simulink model "simulation"  (R2023b)
settings: Solver=VariableStepAuto  StartTime=0.0  StopTime=10.0  RelTol=1e-3
values from neighbouring files (symbols this model uses):
  b1 = b(1,:)    [main.m]    (also in sam_model.m)
  b2 = b(2,:)    [main.m]    (also in sam_model.m)
undefined symbols (not defined in the file or in its folder): a
libraries: fuzblock x2
settings Model: Creator=samee  LastModifiedBy=srd2

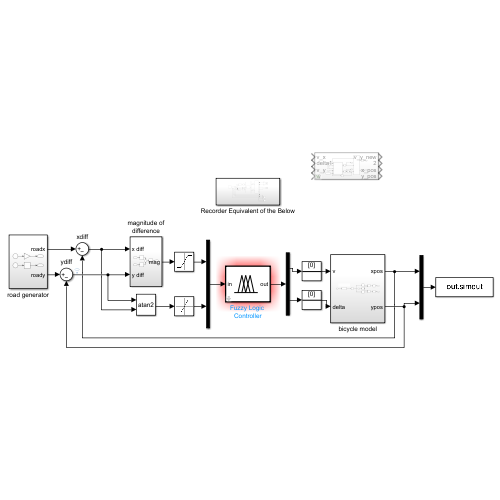
[thumbnail: Simulink's stored preview of the top-level diagram]
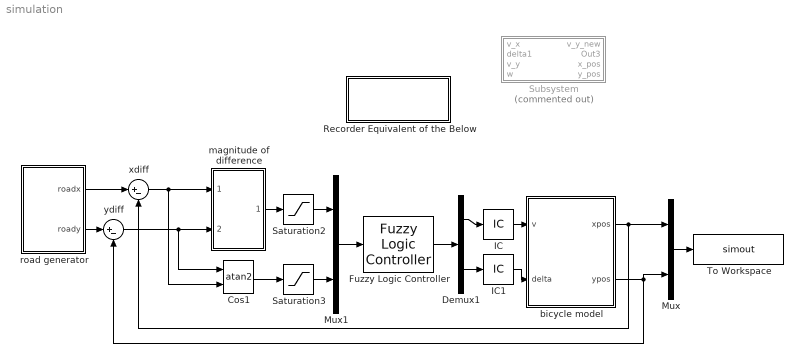
== system simulation ==
  Cos1 : Trigonometry  Operator=atan2
  Demux1 : Demux  Outputs=2
  Fuzzy Logic Controller : fuzblock/Fuzzy Logic  Controller  FIS=fis  OutputSampleNumber=101  DataType=double  FuzzifiedInputs=off  RuleFiringStrengths=off  RuleOutputs=off  AggregatedOutputs=off  SimulateUsing=Interpreted execution  OutOfRangeInputValueMessage=warning  NoRuleFiredMessage=warning  EmptyOutputFuzzySetMessage=warning
  IC : InitialCondition  Value=0
  IC1 : InitialCondition  Value=0
  Mux : Mux  Inputs=2
  Mux1 : Mux  Inputs=2
  Recorder Equivalent of the Below : Subsystem
  Saturation2 : Saturate  UpperLimit=5  LowerLimit=0  LinearizeAsGain=off
  Saturation3 : Saturate  UpperLimit=1  LowerLimit=-1
  Subsystem : Subsystem  Commented=on
  To Workspace : ToWorkspace  VariableName=simout  SaveFormat=Timeseries  SampleTime=-1
  bicycle model : Subsystem
  magnitude of difference : Subsystem
  road generator : Subsystem
  xdiff : Sum  Inputs=|+-
  ydiff : Sum  Inputs=|+-
  wires:
  Saturation2/1 -> Mux1/1
  Fuzzy Logic Controller/1 -> Demux1/1
  Demux1/2 -> IC1/1
  ydiff/1 -> Cos1/1, magnitude of difference/2(y diff)
  Mux1/1 -> Fuzzy Logic Controller/1
  road generator/2(roady) -> ydiff/1
  road generator/1(roadx) -> xdiff/1
  Demux1/1 -> IC/1
  IC1/1 -> bicycle model/2(delta)
  magnitude of difference/1(mag) -> Saturation2/1
  Saturation3/1 -> Mux1/2
  bicycle model/1(xpos) -> Mux/1, xdiff/2
  Cos1/1 -> Saturation3/1
  xdiff/1 -> Cos1/2, magnitude of difference/1(x diff)
  IC/1 -> bicycle model/1(v)
  bicycle model/2(ypos) -> Mux/2, ydiff/2
  Mux/1 -> To Workspace/1

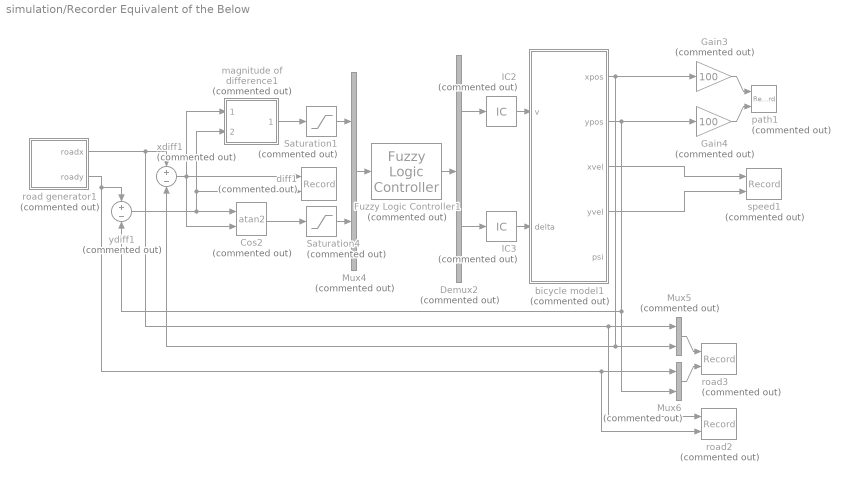
== system simulation/Recorder Equivalent of the Below ==
  Cos2 : Trigonometry  Commented=on  Operator=atan2
  Demux2 : Demux  Commented=on  Outputs=2
  Fuzzy Logic Controller1 : fuzblock/Fuzzy Logic  Controller  Commented=on  FIS=fis  OutputSampleNumber=101  DataType=double  FuzzifiedInputs=off  RuleFiringStrengths=off  RuleOutputs=off  AggregatedOutputs=off  SimulateUsing=Interpreted execution  OutOfRangeInputValueMessage=warning  NoRuleFiredMessage=warning  EmptyOutputFuzzySetMessage=warning
  Gain3 : Gain  Commented=on  Gain=100
  Gain4 : Gain  Commented=on  Gain=100
  IC2 : InitialCondition  Commented=on  Value=0
  IC3 : InitialCondition  Commented=on  Value=0
  Mux4 : Mux  Commented=on  Inputs=2
  Mux5 : Mux  Commented=on  Inputs=2
  Mux6 : Mux  Commented=on  Inputs=2
  Saturation1 : Saturate  Commented=on  UpperLimit=100  LowerLimit=0  LinearizeAsGain=off
  Saturation4 : Saturate  Commented=on  UpperLimit=1  LowerLimit=-1
  bicycle model1 : Subsystem  Commented=on
  diff1 : Record  Commented=on  FileSettingsInternal="{\"entries\":[{\"content\":{\"excelSettings\":{\"content\":{},\"type\":\"Streamout.ExcelSettings\"}},\"type\":\"Streamout.FileSettingStorage\",\"uuid\":\"\"}],\"packageUris\":[\"http:\\/\\/schema.mathworks.com\\/mf0\\/streamout_blocks\\/R2020a\"],\"version\":\"1.0\"}"  Layout=[1 1]  SignalsInternal="{\"entries\":[{\"content\":{\"signals\":[{\"content\":{\"blockPath\":[],\"dimensions\":[1],\"domain\":\"\",\"lineColor\":\"#edb120\",\"plots\":[1],\"port\":1,\"signalID\":48,\"signalName\":\"xdiff\"},\"type\":\"RecordBlkView.Signal\",\"uuid\":\"\"},{\"content\":{\"blockPath\":[],\"dimensions\":[1],\"domain\":\"\",\"lineColor\":\"#7e2f8e\",\"plots\":[1],\"port\":2,\"signalID\":51,\"signalName\":\"ydiff\"},\"type\":\"RecordBlkView.Signal\",\"uuid\":\"\"}]},\"type\":\"RecordBlkView.InputSignals\",\"uuid\":\"\"}],\"packageUris\":[\"http:\\/\\/schema.mathworks.com\\/mf0\\/streamout_blocks\\/R2020a\"],\"version\":\"1.0\"}"  VisualizationBindings="{\"xyplotplugin\":{\"info\":[{\"series\":[{\"bindingParametersList\":[{\"parameter\":\"X-Axis\",\"signalID\":48,\"signalName\":\"xdiff\"},{\"parameter\":\"Y-Axis\",\"signalID\":51,\"signalName\":\"ydiff\"}],\"seriesID\":23733}],\"subplotID\":1}]}}"  CompatibilityTag=XY
  magnitude of difference1 : Subsystem  Commented=on
  path1 : Record  Commented=on  FileSettingsInternal="{\"entries\":[{\"content\":{\"excelSettings\":{\"content\":{},\"type\":\"Streamout.ExcelSettings\"}},\"type\":\"Streamout.FileSettingStorage\",\"uuid\":\"\"}],\"packageUris\":[\"http:\\/\\/schema.mathworks.com\\/mf0\\/streamout_blocks\\/R2020a\"],\"version\":\"1.0\"}"  Layout=[1 1]  SignalsInternal="{\"entries\":[{\"content\":{\"signals\":[{\"content\":{\"blockPath\":[],\"dimensions\":[1],\"domain\":\"\",\"lineColor\":\"#77ac30\",\"plots\":[1],\"port\":1,\"signalID\":40,\"signalName\":\"Gain\"},\"type\":\"RecordBlkView.Signal\",\"uuid\":\"\"},{\"content\":{\"blockPath\":[],\"dimensions\":[1],\"domain\":\"\",\"lineColor\":\"#4dbeee\",\"plots\":[1],\"port\":2,\"signalID\":43,\"signalName\":\"Gain1\"},\"type\":\"RecordBlkView.Signal\",\"uuid\":\"\"}]},\"type\":\"RecordBlkView.InputSignals\",\"uuid\":\"\"}],\"packageUris\":[\"http:\\/\\/schema.mathworks.com\\/mf0\\/streamout_blocks\\/R2020a\"],\"version\":\"1.0\"}"  VisualizationBindings="{\"xyplotplugin\":{\"info\":[{\"series\":[{\"bindingParametersList\":[{\"parameter\":\"X-Axis\",\"signalID\":40,\"signalName\":\"Gain\"},{\"parameter\":\"Y-Axis\",\"signalID\":43,\"signalName\":\"Gain1\"}],\"seriesID\":21120}],\"subplotID\":1}]}}"  CompatibilityTag=XY
  road generator1 : Subsystem  Commented=on
  road2 : Record  Commented=on  FileSettingsInternal="{\"entries\":[{\"content\":{\"excelSettings\":{\"content\":{},\"type\":\"Streamout.ExcelSettings\"}},\"type\":\"Streamout.FileSettingStorage\",\"uuid\":\"\"}],\"packageUris\":[\"http:\\/\\/schema.mathworks.com\\/mf0\\/streamout_blocks\\/R2020a\"],\"version\":\"1.0\"}"  Layout=[1 1]  SignalsInternal="{\"entries\":[{\"content\":{\"signals\":[{\"content\":{\"blockPath\":[],\"dimensions\":[1],\"domain\":\"\",\"lineColor\":\"#a2142f\",\"plots\":[1],\"port\":1,\"signalID\":32,\"signalName\":\"road generator:1\"},\"type\":\"RecordBlkView.Signal\",\"uuid\":\"\"},{\"content\":{\"blockPath\":[],\"dimensions\":[1],\"domain\":\"\",\"lineColor\":\"#139fff\",\"plots\":[1],\"port\":2,\"signalID\":35,\"signalName\":\"road generator:2\"},\"type\":\"RecordBlkView.Signal\",\"uuid\":\"\"}]},\"type\":\"RecordBlkView.InputSignals\",\"uuid\":\"\"}],\"packageUris\":[\"http:\\/\\/schema.mathworks.com\\/mf0\\/streamout_blocks\\/R2020a\"],\"version\":\"1.0\"}"  VisualizationBindings="{\"xyplotplugin\":{\"info\":[{\"series\":[{\"bindingParametersList\":[{\"parameter\":\"X-Axis\",\"signalID\":32,\"signalName\":\"road generator:1\"},{\"parameter\":\"Y-Axis\",\"signalID\":35,\"signalName\":\"road generator:2\"}],\"seriesID\":48995}],\"subplotID\":1}]}}"  CompatibilityTag=XY
  road3 : Record  Commented=on  FileSettingsInternal="{\"entries\":[{\"content\":{\"excelSettings\":{\"content\":{},\"type\":\"Streamout.ExcelSettings\"}},\"type\":\"Streamout.FileSettingStorage\",\"uuid\":\"\"}],\"packageUris\":[\"http:\\/\\/schema.mathworks.com\\/mf0\\/streamout_blocks\\/R2020a\"],\"version\":\"1.0\"}"  Layout=[1 1]  SignalsInternal="{\"entries\":[{\"content\":{\"signals\":[{\"content\":{\"blockPath\":[],\"dimensions\":[2],\"domain\":\"\",\"hasChildren\":true,\"lineColor\":\"#a2142f\",\"port\":1,\"signalID\":16,\"signalName\":\"Mux1\"},\"type\":\"RecordBlkView.Signal\",\"uuid\":\"\"},{\"content\":{\"blockPath\":[],\"channel\":[1],\"dimensions\":[2],\"domain\":\"\",\"lineColor\":\"#139fff\",\"parentID\":16,\"plots\":[1],\"port\":1,\"signalID\":17,\"signalName\":\"Mux1\"},\"type\":\"RecordBlkView.Signal\",\"uuid\":\"\"},{\"content\":{\"blockPath\":[],\"channel\":[2],\"dimensions\":[2],\"domain\":\"\",\"lineColor\":\"#fe330a\",\"parentID\":16,\"plots\":[1],\"port\":1,\"signalID\":18,\"signalName\":\"Mux1\"},\"type\":\"RecordBlkView.Signal\",\"uuid\":\"\"},{\"content\":{\"blockPath\":[],\"dimensions\":[2],\"domain\":\"\",\"hasChildren\":true,\"lineColor\":\"#ff6929\",\"port\":2,\"signalID\":23,\"signalName\":\"Mux2\"},\"type\":\"RecordBlkView.Signal\",\"uuid\":\"\"},{\"content\":{\"blockPath\":[],\"channel\":[1],\"dimensions\":[2],\"domain\":\"\",\"lineColor\":\"#b746ff\",\"parentID\":23,\"plots\":[1],\"port\":2,\"signalID\":24,\"signalName\":\"Mux2\"},\"type\":\"RecordBlkView.Signal\",\"uuid\":\"\"},{\"content\":{\"blockPath\":[],\"channel\":[2],\"dimensions\":[2],\"domain\":\"\",\"lineColor\":\"#22b573\",\"parentID\":23,\"plots\":[1],\"port\":2,\"signalID\":25,\"signalName\":\"Mux2\"},\"type\":\"RecordBlkView.Signal\",\"uuid\":\"\"}]},\"type\":\"RecordBlkView.InputSignals\",\"uuid\":\"\"}],\"packageUris\":[\"http:\\/\\/schema.mathworks.com\\/mf0\\/streamout_blocks\\/R2020a\"],\"version\":\"1.0\"}"  VisualizationBindings="{\"xyplotplugin\":{\"info\":[{\"series\":[{\"bindingParametersList\":[{\"parameter\":\"X-Axis\",\"signalID\":17,\"signalName\":\"Mux1(1)\"},{\"parameter\":\"Y-Axis\",\"signalID\":25,\"signalName\":\"Mux2(2)\"}],\"seriesID\":7025},{\"bindingParametersList\":[{\"parameter\":\"X-Axis\",\"signalID\":18,\"signalName\":\"Mux1(2)\"},{\"parameter\":\"Y-Axis\",\"signalID\":24,\"signalName\":\"Mux2(1)\"}],\"seriesID\":49155}],\"subplotID\":1}]}}"  CompatibilityTag=XY
  speed1 : Record  Commented=on  FileSettingsInternal="{\"entries\":[{\"content\":{\"excelSettings\":{\"content\":{},\"type\":\"Streamout.ExcelSettings\"}},\"type\":\"Streamout.FileSettingStorage\",\"uuid\":\"\"}],\"packageUris\":[\"http:\\/\\/schema.mathworks.com\\/mf0\\/streamout_blocks\\/R2020a\"],\"version\":\"1.0\"}"  Layout=[1 1]  SignalsInternal="{\"entries\":[{\"content\":{\"signals\":[{\"content\":{\"blockPath\":[],\"dimensions\":[1],\"domain\":\"\",\"lineColor\":\"#ff6929\",\"plots\":[1],\"port\":1,\"signalID\":8,\"signalName\":\"bicycle model:3\"},\"type\":\"RecordBlkView.Signal\",\"uuid\":\"\"},{\"content\":{\"blockPath\":[],\"dimensions\":[1],\"domain\":\"\",\"lineColor\":\"#b746ff\",\"plots\":[1],\"port\":2,\"signalID\":11,\"signalName\":\"bicycle model:4\"},\"type\":\"RecordBlkView.Signal\",\"uuid\":\"\"}]},\"type\":\"RecordBlkView.InputSignals\",\"uuid\":\"\"}],\"packageUris\":[\"http:\\/\\/schema.mathworks.com\\/mf0\\/streamout_blocks\\/R2020a\"],\"version\":\"1.0\"}"  VisualizationBindings="{\"xyplotplugin\":{\"info\":[{\"series\":[{\"bindingParametersList\":[{\"parameter\":\"X-Axis\",\"signalID\":8,\"signalName\":\"bicycle model:3\"},{\"parameter\":\"Y-Axis\",\"signalID\":11,\"signalName\":\"bicycle model:4\"}],\"seriesID\":3598}],\"subplotID\":1}]}}"  CompatibilityTag=XY
  xdiff1 : Sum  Commented=on  Inputs=+-
  ydiff1 : Sum  Commented=on  Inputs=+-
  wires:
  Gain3/1 -> path1/1
  road generator1/1(roadx) -> xdiff1/1, Mux5/1, road2/1
  Cos2/1 -> Saturation4/1
  Fuzzy Logic Controller1/1 -> Demux2/1
  bicycle model1/1(xpos) -> Gain3/1, xdiff1/2, Mux5/2
  bicycle model1/2(ypos) -> Gain4/1, Mux6/2, ydiff1/2
  ydiff1/1 -> magnitude of difference1/2(y diff), diff1/2, Cos2/1
  Mux4/1 -> Fuzzy Logic Controller1/1
  Demux2/1 -> IC2/1
  Mux5/1 -> road3/1
  Saturation1/1 -> Mux4/1
  magnitude of difference1/1(mag) -> Saturation1/1
  IC3/1 -> bicycle model1/2(delta)
  bicycle model1/4(yvel) -> speed1/2
  bicycle model1/3(xvel) -> speed1/1
  Gain4/1 -> path1/2
  Mux6/1 -> road3/2
  Saturation4/1 -> Mux4/2
  xdiff1/1 -> Cos2/2, diff1/1, magnitude of difference1/1(x diff)
  Demux2/2 -> IC3/1
  road generator1/2(roady) -> road2/2, Mux6/1, ydiff1/1
  IC2/1 -> bicycle model1/1(v)

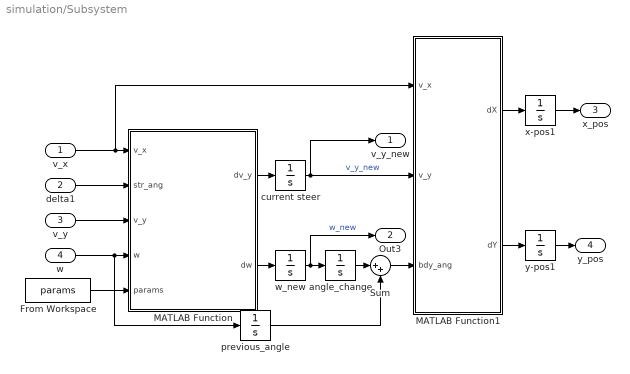
== system simulation/Subsystem ==
  v_x : Inport
  delta1 : Inport  Port=2  OutDataTypeStr=double
  v_y : Inport  Port=3
  w : Inport  Port=4
  From Workspace : FromWorkspace  VariableName=params
  MATLAB Function : MATLAB Function  TreatAsAtomicUnit=on
  MATLAB Function1 : MATLAB Function  TreatAsAtomicUnit=on
  Sum : Sum  Inputs=|++
  angle_change : Integrator
  current steer : Integrator
  previous_angle : Integrator
  w_new : Integrator
  x-pos1 : Integrator
  y-pos1 : Integrator
  v_y_new : Outport
  Out3 : Outport  Port=2
  x_pos : Outport  Port=3
  y_pos : Outport  Port=4
  wires:
  previous_angle/1 -> Sum/2
  w_new/1 -> Out3/1, angle_change/1  "w_new"
  angle_change/1 -> Sum/1
  v_y/1 -> MATLAB Function/3(v_y)
  MATLAB Function1/1(dX) -> x-pos1/1
  MATLAB Function/1(dv_y) -> current steer/1
  MATLAB Function/2(dw) -> w_new/1
  From Workspace/1 -> MATLAB Function/5(params)
  Sum/1 -> MATLAB Function1/3(bdy_ang)
  MATLAB Function1/2(dY) -> y-pos1/1
  v_x/1 -> MATLAB Function1/1(v_x), MATLAB Function/1(v_x)
  delta1/1 -> MATLAB Function/2(str_ang)
  w/1 -> previous_angle/1, MATLAB Function/4(w)
  current steer/1 -> MATLAB Function1/2(v_y), v_y_new/1  "v_y_new"
  y-pos1/1 -> y_pos/1
  x-pos1/1 -> x_pos/1

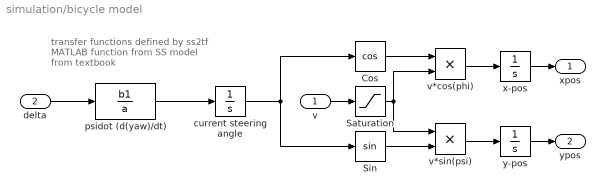
== system simulation/bicycle model ==
  note: transfer functions defined by ss2tf
      | MATLAB function from SS model
      | from textbook
  v : Inport
  delta : Inport  Port=2  OutDataTypeStr=double
  Cos : Trigonometry  Operator=cos
  Saturation : Saturate  UpperLimit=30  LowerLimit=-30
  Sin : Trigonometry
  current steering angle : Integrator
  psidot (d(yaw)/dt) : TransferFcn  Numerator=b1  Denominator=a  ParameterTunability=Optimized  ContinuousStateAttributes='psidot'
  v*cos(phi) : Product
  v*sin(psi) : Product
  x-pos : Integrator
  y-pos : Integrator
  xpos : Outport
  ypos : Outport  Port=2
  wires:
  psidot (d(yaw)/dt)/1 -> current steering angle/1
  v*sin(psi)/1 -> y-pos/1
  current steering angle/1 -> Sin/1, Cos/1
  delta/1 -> psidot (d(yaw)/dt)/1
  Sin/1 -> v*sin(psi)/2
  v*cos(phi)/1 -> x-pos/1
  Cos/1 -> v*cos(phi)/1
  y-pos/1 -> ypos/1
  x-pos/1 -> xpos/1
  Saturation/1 -> v*cos(phi)/2, v*sin(psi)/1
  v/1 -> Saturation/1

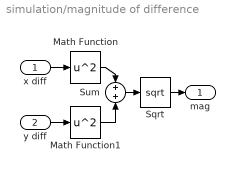
== system simulation/magnitude of difference ==
  x diff : Inport
  y diff : Inport  Port=2
  Math Function : Math  Operator=square
  Math Function1 : Math  Operator=square
  Sqrt : Sqrt
  Sum : Sum  Inputs=+|+
  mag : Outport
  wires:
  Math Function/1 -> Sum/1
  Sum/1 -> Sqrt/1
  Math Function1/1 -> Sum/2
  y diff/1 -> Math Function1/1
  Sqrt/1 -> mag/1
  x diff/1 -> Math Function/1

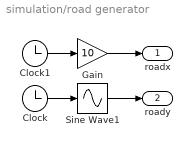
== system simulation/road generator ==
  Clock : Clock
  Clock1 : Clock
  Gain : Gain  Gain=10
  Sine Wave1 : Sin  TimeSource=Use external signal  Amplitude=10  Frequency=0.05  Phase=1  SampleTime=0
  roadx : Outport
  roady : Outport  Port=2
  wires:
  Clock/1 -> Sine Wave1/1
  Sine Wave1/1 -> roady/1
  Clock1/1 -> Gain/1
  Gain/1 -> roadx/1

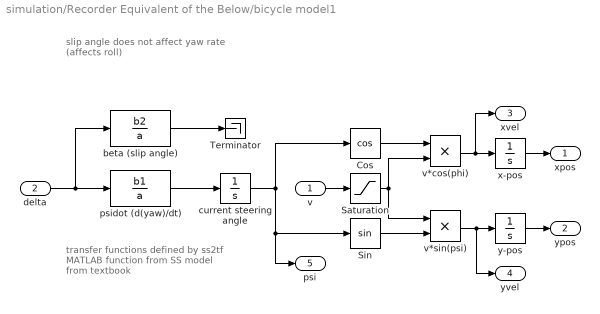
== system simulation/Recorder Equivalent of the Below/bicycle model1 ==
  note: transfer functions defined by ss2tf
      | MATLAB function from SS model
      | from textbook
  note: slip angle does not affect yaw rate
      | (affects roll)
  v : Inport
  delta : Inport  Port=2  OutDataTypeStr=double
  Cos : Trigonometry  Operator=cos
  Saturation : Saturate  UpperLimit=30  LowerLimit=-30
  Sin : Trigonometry
  Terminator : Terminator
  beta (slip angle) : TransferFcn  Numerator=b2  Denominator=a  ContinuousStateAttributes='beta'
  current steering angle : Integrator
  psidot (d(yaw)/dt) : TransferFcn  Numerator=b1  Denominator=a  ParameterTunability=Optimized  ContinuousStateAttributes='psidot'
  v*cos(phi) : Product
  v*sin(psi) : Product
  x-pos : Integrator
  y-pos : Integrator
  xpos : Outport
  ypos : Outport  Port=2
  xvel : Outport  Port=3
  yvel : Outport  Port=4
  psi : Outport  Port=5
  wires:
  psidot (d(yaw)/dt)/1 -> current steering angle/1
  v*sin(psi)/1 -> y-pos/1, yvel/1
  current steering angle/1 -> psi/1, Sin/1, Cos/1
  delta/1 -> psidot (d(yaw)/dt)/1, beta (slip angle)/1
  Sin/1 -> v*sin(psi)/2
  v*cos(phi)/1 -> x-pos/1, xvel/1
  Cos/1 -> v*cos(phi)/1
  y-pos/1 -> ypos/1
  x-pos/1 -> xpos/1
  Saturation/1 -> v*cos(phi)/2, v*sin(psi)/1
  v/1 -> Saturation/1
  beta (slip angle)/1 -> Terminator/1

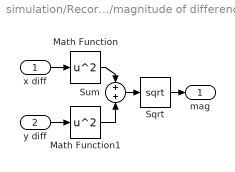
== system simulation/Recorder Equivalent of the Below/magnitude of difference1 ==
  x diff : Inport
  y diff : Inport  Port=2
  Math Function : Math  Operator=square
  Math Function1 : Math  Operator=square
  Sqrt : Sqrt
  Sum : Sum  Inputs=+|+
  mag : Outport
  wires:
  Math Function/1 -> Sum/1
  Sum/1 -> Sqrt/1
  Math Function1/1 -> Sum/2
  y diff/1 -> Math Function1/1
  Sqrt/1 -> mag/1
  x diff/1 -> Math Function/1

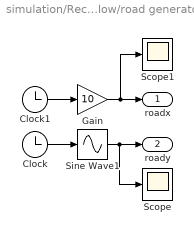
== system simulation/Recorder Equivalent of the Below/road generator1 ==
  Clock : Clock
  Clock1 : Clock
  Gain : Gain  Gain=10
  Scope : Scope
  Scope1 : Scope
  Sine Wave1 : Sin  TimeSource=Use external signal  Amplitude=10  Frequency=0.05  Phase=1  SampleTime=0
  roadx : Outport
  roady : Outport  Port=2
  wires:
  Clock/1 -> Sine Wave1/1
  Sine Wave1/1 -> Scope/1, roady/1
  Clock1/1 -> Gain/1
  Gain/1 -> roadx/1, Scope1/1

== matlab function simulation/Subsystem/MATLAB Function1 ==
  data: v_x input; v_y input; dX output; bdy_ang input; dY output
function [dX, dY] = new_velocity(v_x, v_y, bdy_ang)
    R_gl = [cos(bdy_ang), sin(bdy_ang);
           -sin(bdy_ang),  cos(bdy_ang)].';
    dV = R_gl * [v_x; v_y];
    
    dX = dV(1); 
    dY = dV(2);
end

== matlab function simulation/Subsystem/MATLAB Function ==
  data: v_x input; str_ang input; v_y input; dv_y output; w input; params input; dw output
function [dv_y, dw] = forward_dynamcis(v_x, str_ang, v_y, w,  params)
    % dv_y = -(car + caf)/(m *v_x) * v_y + (car*lr - caf*lf)/(m *v_x) * w- v_x * w + caf/m * str_ang; 
    % dw     = (car*lr - caf*lf)/(Iz*v_x) * v_y - (car*lr^2 + caf*lf^2)/(Iz*v_x) * w + caf*lf/Iz  * str_ang;
    
    % parameters
    caf = params(1); car = params(2); lf  = params(3); lr  = params(4); 
    m   = params(5); Iz  = params(6);

    % get put equations of kimetmic motion into state space form
    a11 = -(car + caf)/(m *v_x);
    a12 =  (car*lr   -   caf*lf)/(m *v_x) - v_x;
    a21 =  (car*lr   -   caf*lf)/(Iz*v_x);
    a22 = -(car*lr^2 + caf*lf^2)/(Iz*v_x);
    
    b11 = caf/m;
    b21 = caf*lf/Iz;
    
    A = [a11, a12; a21, a22];
    B = [b11; b21];
    
    dX = A * [v_y; w] + B * str_ang;

    dv_y = dX(1); 
    dw = dX(2);
end
